simulink model "simulinkModel"  (R2021a)
settings: Solver=FixedStepDiscrete  StartTime=0.0  StopTime=10.0  RelTol=1e-3
model workspace (MAT data in the model file):
  firstWarning = 1
  originalScenarioChecksum = '9309B486BCEF727DEE1E25828442B4A3'
undefined symbols (not defined in the file or in its folder): driving
libraries: drivingscenarioandsensors x5
(part 1 of 2)
settings Model: Creator=DHEEPAK  LastModifiedBy=DHEEPAK

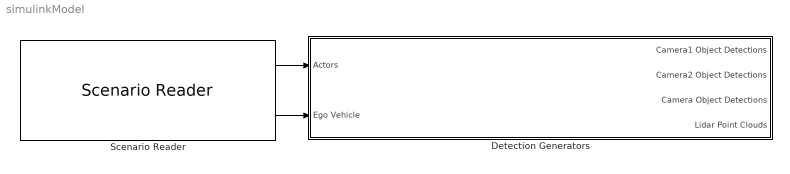
== system simulinkModel ==
  Detection Generators : Subsystem
  Scenario Reader : drivingscenarioandsensors/Scenario Reader  ScenarioSource=From file  ScenarioFileName=D:\1_MATHWORKS_Capstone\1_approachOne\6_unsteadyDriver_Car\scenarioFIile.mat  ScenarioVariableName=scenario  OutputCoordinateSystem=Vehicle coordinates  EgoVehicleSource=Scenario  EgoVehicleActorID=1  OrientVehiclesOnRoad=off  OutputEgoVehiclePose=on  SampleTime=0.1  LaneBoundaryOutput=None  LaneBoundaryDistance=0:0.5:9.5  LaneBoundaryLocation=Center of lane markings  BusNameSource=Auto  BusName=BusActors  BusNumActorsSource=Scenario  BusNumActors=100  BusName2Source=Auto  BusName2=BusLaneBoundaries  BusNumLaneBoundariesSource=Scenario  BusNumLaneBoundaries=10  BusName3Source=Auto  BusName3=BusEgoActor  ShowCoordinateLabels=on  SimulateUsing=Interpreted execution
  wires:
  Scenario Reader/1 -> Detection Generators/1(Actors)
  Scenario Reader/2 -> Detection Generators/2(Ego Vehicle)
